simulink model "nov11"  (R2014a)
settings: Solver=ode45  StartTime=0.0  StopTime=30  FixedStep=0.00001  RelTol=1e-12
values from neighbouring files (symbols this model uses):
  m = [1 t0 (t0)^2 (t0)^3;0 1 (2*(t0)^2) (3*(t0)^2);1 tf (tf)^2 (tf)^3;0 1 (2*(tf)^2) (3*(tf)^2)]    [ControlCinematico.m]    (also in untitled3.m = [1 0 0 0 0 0;0 1 0 0 0 0;0 0 2 0 0 0;1 tf tf^2 tf^3 tf^4 tf^)
libraries: mblibv1 x15
settings Model: Creator=sebastian  LastModifiedBy=root
settings DataIOCC: SignalLoggingSaveFormat=ModelDataLogs
settings DebuggingCC: UnderspecifiedInitializationDetection=Classic  MultiTaskDSMMsg=warning  MultiTaskCondExecSysMsg=none  StateNameClashWarn=warning
settings RTWCC: IncludeERTFirstTime=on
settings SimMechanicsCC: VisOnUpdateDiagram=on  VisDuringSimulation=on

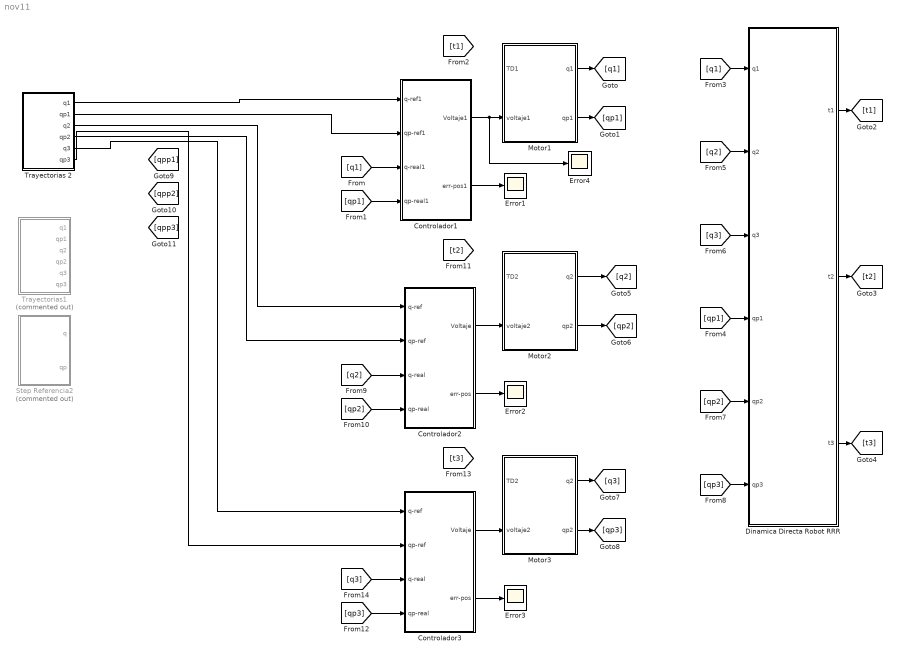
== system nov11 ==
  Controlador1 : Subsystem
  Controlador2 : Subsystem
  Controlador3 : Subsystem
  Dinamica Directa Robot RRR : Subsystem
  Error{1..4} (4 alike) : Scope
      Error1 settings: TimeRange=0.000199999999999978  YMin=-470000  YMax=-455000  SaveName=ScopeData4
      Error2 settings: YMin=0.3178  YMax=0.3188
      Error3 settings: YMin=0.675  YMax=1  SaveName=ScopeData5
      Error4 settings: YMin=-0.12  YMax=0  SaveName=ScopeData12
  Motor1 : Subsystem
  Motor2 : Subsystem
  Motor3 : Subsystem
  Step Referencia2 : Subsystem  Commented=on
  Trayectorias 2 : Subsystem
  Trayectorias1 : Subsystem  Commented=on
  wires:
  Controlador1/1(Voltaje1) -> Error4/1, Motor1/2(voltaje1)
  Controlador1/2(err-pos1) -> Error1/1
  Motor1/1(q1) -> [q1]
  Motor1/2(qp1) -> [qp1]
  Dinamica Directa Robot RRR/1(t1) -> [t1]
  [q1] -> Controlador1/3(q-real1)
  [qp1] -> Controlador1/4(qp-real1)
  [q1] -> Dinamica Directa Robot RRR/1(q1)
  [qp1] -> Dinamica Directa Robot RRR/4(qp1)
  [q2] -> Dinamica Directa Robot RRR/2(q2)
  [q3] -> Dinamica Directa Robot RRR/3(q3)
  [qp2] -> Dinamica Directa Robot RRR/5(qp2)
  [qp3] -> Dinamica Directa Robot RRR/6(qp3)
  Dinamica Directa Robot RRR/2(t2) -> [t2]
  Dinamica Directa Robot RRR/3(t3) -> [t3]
  Controlador2/1(Voltaje) -> Motor2/2(voltaje2)
  Controlador2/2(err-pos) -> Error2/1
  [q2] -> Controlador2/3(q-real)
  [qp2] -> Controlador2/4(qp-real)
  Controlador3/1(Voltaje) -> Motor3/2(voltaje2)
  Controlador3/2(err-pos) -> Error3/1
  Motor3/1(q2) -> [q3]
  Motor3/2(qp2) -> [qp3]
  [q3] -> Controlador3/3(q-real)
  [qp3] -> Controlador3/4(qp-real)
  Motor2/1(q2) -> [q2]
  Motor2/2(qp2) -> [qp2]
  Trayectorias 2/1(q1) -> Controlador1/1(q-ref1)
  Trayectorias 2/2(qp1) -> Controlador1/2(qp-ref1)
  Trayectorias 2/3(q2) -> Controlador2/1(q-ref)
  Trayectorias 2/4(qp2) -> Controlador2/2(qp-ref)
  Trayectorias 2/5(q3) -> Controlador3/1(q-ref)
  Trayectorias 2/6(qp3) -> Controlador3/2(qp-ref)

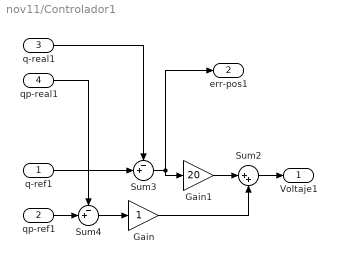
== system nov11/Controlador1 ==
  q-ref1 : Inport
  qp-ref1 : Inport  Port=2
  q-real1 : Inport  Port=3
  qp-real1 : Inport  Port=4
  Gain : Gain
  Gain1 : Gain  Gain=20
  Sum2 : Sum  Inputs=|++
  Sum3 : Sum  Inputs=-+|
  Sum4 : Sum  Inputs=-+|
  Voltaje1 : Outport
  err-pos1 : Outport  Port=2
  wires:
  Gain1/1 -> Sum2/1
  Gain/1 -> Sum2/2
  Sum4/1 -> Gain/1
  Sum2/1 -> Voltaje1/1
  q-ref1/1 -> Sum3/2
  qp-ref1/1 -> Sum4/2
  q-real1/1 -> Sum3/1
  qp-real1/1 -> Sum4/1
  Sum3/1 -> Gain1/1, err-pos1/1

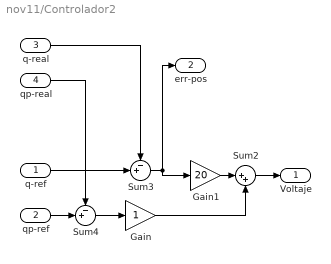
== system nov11/Controlador2 ==
  q-ref : Inport
  qp-ref : Inport  Port=2
  q-real : Inport  Port=3
  qp-real : Inport  Port=4
  Gain : Gain
  Gain1 : Gain  Gain=20
  Sum2 : Sum  Inputs=|++
  Sum3 : Sum  Inputs=-+|
  Sum4 : Sum  Inputs=-+|
  Voltaje : Outport
  err-pos : Outport  Port=2
  wires:
  Gain1/1 -> Sum2/1
  Gain/1 -> Sum2/2
  Sum4/1 -> Gain/1
  Sum2/1 -> Voltaje/1
  q-ref/1 -> Sum3/2
  qp-ref/1 -> Sum4/2
  q-real/1 -> Sum3/1
  qp-real/1 -> Sum4/1
  Sum3/1 -> Gain1/1, err-pos/1

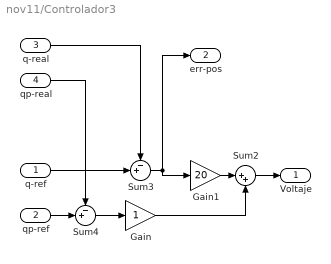
== system nov11/Controlador3 ==
  q-ref : Inport
  qp-ref : Inport  Port=2
  q-real : Inport  Port=3
  qp-real : Inport  Port=4
  Gain : Gain
  Gain1 : Gain  Gain=20
  Sum2 : Sum  Inputs=|++
  Sum3 : Sum  Inputs=-+|
  Sum4 : Sum  Inputs=-+|
  Voltaje : Outport
  err-pos : Outport  Port=2
  wires:
  Gain1/1 -> Sum2/1
  Gain/1 -> Sum2/2
  Sum4/1 -> Gain/1
  Sum2/1 -> Voltaje/1
  q-ref/1 -> Sum3/2
  qp-ref/1 -> Sum4/2
  q-real/1 -> Sum3/1
  qp-real/1 -> Sum4/1
  Sum3/1 -> Gain1/1, err-pos/1

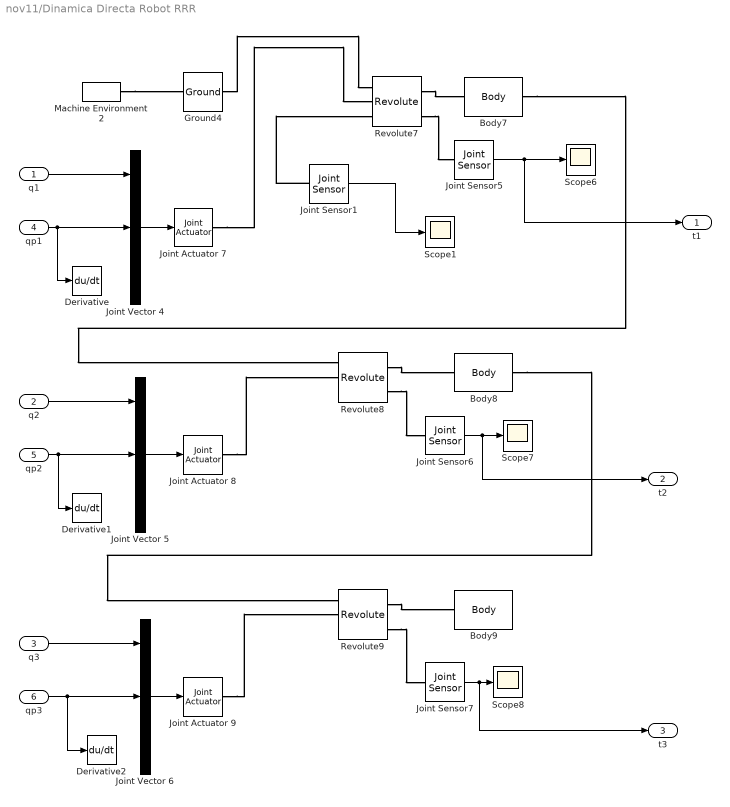
== system nov11/Dinamica Directa Robot RRR ==
  q1 : Inport
  q2 : Inport  Port=2
  q3 : Inport  Port=3
  qp1 : Inport  Port=4
  qp2 : Inport  Port=5
  qp3 : Inport  Port=6
  Body7 : mblibv1/Bodies/Body  LConnTagsString=CS1  RConnTagsString=CS2  UpdateFromCAD=off  DialogClass=MechanicalBodyBlock  Mass=1  MassUnits=kg  InertiaUnits=kg*m^2  Inertia=[0 0 0;0 0 0;0 0 33.3333]  Shape=Cylinder  ShapeDims=[1 1]  ShapeUnits=m  ShapeUse=false  Density=1  DensityUnits=kg/m^3  DensityUse=false  GraphicsMode=MACHINE_DEFAULT  BodyColorSelMode=COLORPALETTE  BodyColor=[0 1 0]  AttachedToCS=CG  CG=Left$CG$[0 10 0]$WORLD$WORLD$m$[0 0 0]$Euler X-Y-Z$deg$WORLD$false$none  WorkingFrames=Left$CS1$[0 0 0]$World$World$m$[0 0 0]$Euler X-Y-Z$deg$WORLD$true$none#Right$CS2$[0 20 0]$World$World$m$[0 0 0]$Euler X-Y-Z$deg$WORLD$true$none  CGPos=[0 10 0]  CGRot=[0 0 0]  CS0Pos=[]  CS0Rot=[]  CS1Pos=[0 0 0]  CS1Rot=[0 0 0]  CS2Pos=[0 20 0]  CS2Rot=[0 0 0]  CS3Pos=[]  CS3Rot=[]  CS4Pos=[]  CS4Rot=[]  CS5Pos=[]  CS5Rot=[]  CS6Pos=[]  CS6Rot=[]  CS7Pos=[]  CS7Rot=[]  CS8Pos=[]  CS8Rot=[]  CS9Pos=[]  CS9Rot=[]  CS10Pos=[]  CS10Rot=[]  CS11Pos=[]  CS11Rot=[]  CS12Pos=[]  CS12Rot=[]  CS13Pos=[]  CS13Rot=[]  CS14Pos=[]  CS14Rot=[]  CS15Pos=[]  CS15Rot=[]  CS16Pos=[]  CS16Rot=[]  CS17Pos=[]  CS17Rot=[]  CS18Pos=[]  CS18Rot=[]  CS19Pos=[]  CS19Rot=[]  CS20Pos=[]  CS20Rot=[]
  Body8 : mblibv1/Bodies/Body  LConnTagsString=CS1  RConnTagsString=CS2  UpdateFromCAD=off  DialogClass=MechanicalBodyBlock  Mass=1  MassUnits=kg  InertiaUnits=kg*m^2  Inertia=[0 0 0;0 0 0;0 0 33.3333]  Shape=Cylinder  ShapeDims=[1 1]  ShapeUnits=m  ShapeUse=false  Density=1  DensityUnits=kg/m^3  DensityUse=false  GraphicsMode=MACHINE_DEFAULT  BodyColorSelMode=COLORPALETTE  BodyColor=[0 1 0]  AttachedToCS=CG  CG=Left$CG$[10 20 0]$WORLD$WORLD$m$[0 0 0]$Euler X-Y-Z$deg$WORLD$false$none  WorkingFrames=Left$CS1$[0 20 0]$World$World$m$[0 0 0]$Euler X-Y-Z$deg$WORLD$true$none#Right$CS2$[20 20 0]$World$World$m$[0 0 0]$Euler X-Y-Z$deg$WORLD$true$none  CGPos=[10 20 0]  CGRot=[0 0 0]  CS0Pos=[]  CS0Rot=[]  CS1Pos=[0 20 0]  CS1Rot=[0 0 0]  CS2Pos=[20 20 0]  CS2Rot=[0 0 0]  CS3Pos=[]  CS3Rot=[]  CS4Pos=[]  CS4Rot=[]  CS5Pos=[]  CS5Rot=[]  CS6Pos=[]  CS6Rot=[]  CS7Pos=[]  CS7Rot=[]  CS8Pos=[]  CS8Rot=[]  CS9Pos=[]  CS9Rot=[]  CS10Pos=[]  CS10Rot=[]  CS11Pos=[]  CS11Rot=[]  CS12Pos=[]  CS12Rot=[]  CS13Pos=[]  CS13Rot=[]  CS14Pos=[]  CS14Rot=[]  CS15Pos=[]  CS15Rot=[]  CS16Pos=[]  CS16Rot=[]  CS17Pos=[]  CS17Rot=[]  CS18Pos=[]  CS18Rot=[]  CS19Pos=[]  CS19Rot=[]  CS20Pos=[]  CS20Rot=[]
  Body9 : mblibv1/Bodies/Body  LConnTagsString=CS1  RConnTagsString=CS2  UpdateFromCAD=off  DialogClass=MechanicalBodyBlock  Mass=1  MassUnits=kg  InertiaUnits=kg*m^2  Inertia=[0 0 0;0 0 0;0 0 8.3333]  Shape=Cylinder  ShapeDims=[1 1]  ShapeUnits=m  ShapeUse=false  Density=1  DensityUnits=kg/m^3  DensityUse=false  GraphicsMode=MACHINE_DEFAULT  BodyColorSelMode=COLORPALETTE  BodyColor=[0 1 0]  AttachedToCS=CG  CG=Left$CG$[20 15 0]$WORLD$WORLD$m$[0 0 0]$Euler X-Y-Z$deg$WORLD$false$none  WorkingFrames=Left$CS1$[20 20 0]$World$World$m$[0 0 0]$Euler X-Y-Z$deg$WORLD$true$none#Right$CS2$[20 10 0]$World$World$m$[0 0 0]$Euler X-Y-Z$deg$WORLD$true$none  CGPos=[20 15 0]  CGRot=[0 0 0]  CS0Pos=[]  CS0Rot=[]  CS1Pos=[20 20 0]  CS1Rot=[0 0 0]  CS2Pos=[20 10 0]  CS2Rot=[0 0 0]  CS3Pos=[]  CS3Rot=[]  CS4Pos=[]  CS4Rot=[]  CS5Pos=[]  CS5Rot=[]  CS6Pos=[]  CS6Rot=[]  CS7Pos=[]  CS7Rot=[]  CS8Pos=[]  CS8Rot=[]  CS9Pos=[]  CS9Rot=[]  CS10Pos=[]  CS10Rot=[]  CS11Pos=[]  CS11Rot=[]  CS12Pos=[]  CS12Rot=[]  CS13Pos=[]  CS13Rot=[]  CS14Pos=[]  CS14Rot=[]  CS15Pos=[]  CS15Rot=[]  CS16Pos=[]  CS16Rot=[]  CS17Pos=[]  CS17Rot=[]  CS18Pos=[]  CS18Rot=[]  CS19Pos=[]  CS19Rot=[]  CS20Pos=[]  CS20Rot=[]
  Derivative : Derivative
  Derivative1 : Derivative
  Derivative2 : Derivative
  Ground4 : mblibv1/Bodies/Ground  UpdateFromCAD=off  LeftPortType=env  RightPortType=workingframe  PhysicalDomain=Mechanical  DialogClass=GroundBlock  CoordPosition=[0 0 0]  CoordPositionUnits=m  StateVectorMgrId=1  MachineId=[2 0]  ShowEnvPort=on  ParameterChecksum=[821500782, 2772552656, 1304883052, 3709367703]  TopologyChecksum=[4015144124, 1642793208, 2502497068, 3913265325]
  Joint Actuator 7 : mblibv1/Sensors &  Actuators/Joint Actuator  UpdateFromCAD=off  PhysicalDomain=Mechanical  PortType=blob  ActuationStyle=Motion  AngleUnits=rad  ArcVelocityUnits=rad/s  ArcAccelerationUnits=rad/s^2  CoordPositionUnits=m  VelocityUnits=m/s  AccelerationUnits=m/s^2  ForceUnits=N  TorqueUnits=N*m  ActiveIO=on  Width=3  DialogClass=MechanicalActuatorBlock  Primitive=R1  ReferenceFrame=Absolute (World)
  Joint Actuator 8 : mblibv1/Sensors &  Actuators/Joint Actuator  UpdateFromCAD=off  PhysicalDomain=Mechanical  PortType=blob  ActuationStyle=Motion  AngleUnits=rad  ArcVelocityUnits=rad/s  ArcAccelerationUnits=rad/s^2  CoordPositionUnits=m  VelocityUnits=m/s  AccelerationUnits=m/s^2  ForceUnits=N  TorqueUnits=N*m  ActiveIO=on  Width=3  DialogClass=MechanicalActuatorBlock  Primitive=R1  ReferenceFrame=Absolute (World)
  Joint Actuator 9 : mblibv1/Sensors &  Actuators/Joint Actuator  UpdateFromCAD=off  PhysicalDomain=Mechanical  PortType=blob  ActuationStyle=Motion  AngleUnits=rad  ArcVelocityUnits=rad/s  ArcAccelerationUnits=rad/s^2  CoordPositionUnits=m  VelocityUnits=m/s  AccelerationUnits=m/s^2  ForceUnits=N  TorqueUnits=N*m  ActiveIO=on  Width=3  DialogClass=MechanicalActuatorBlock  Primitive=R1  ReferenceFrame=Absolute (World)
  Joint Sensor1 : mblibv1/Sensors &  Actuators/Joint Sensor  UpdateFromCAD=off  PhysicalDomain=Mechanical  PortType=blob  Muxed=on  Pose=off  Angle=on  AngleUnits=rad  ArcVelocity=off  ArcVelocityUnits=deg/s  ArcAcceleration=off  ArcAccelerationUnits=deg/s^2  CoordPosition=on  CoordPositionUnits=m  Velocity=off  VelocityUnits=m/s  Acceleration=off  AccelerationUnits=m/s^2  Quaternion=on  QuaternionDT=off  QuaternionDDT=off  QuaternionUnits=off  OutputVector=[1]  ActiveIO=on  Width=1  DialogClass=MechanicalSensorBlock  Primitive=R1  Force=off  ForceUnits=N  Torque=off  TorqueUnits=N*m  ReferenceFrame=Absolute (World)  ReactionSensedSide=Follower  ReactionReferenceFrame=Absolute (World)  ReactionForce=off  ReactionForceUnits=N  ReactionMoment=off  ReactionMomentUnits=N*m
  Joint Sensor5 : mblibv1/Sensors &  Actuators/Joint Sensor  UpdateFromCAD=off  PhysicalDomain=Mechanical  PortType=blob  Muxed=on  Pose=off  Angle=off  AngleUnits=deg  ArcVelocity=off  ArcVelocityUnits=deg/s  ArcAcceleration=off  ArcAccelerationUnits=deg/s^2  CoordPosition=on  CoordPositionUnits=m  Velocity=off  VelocityUnits=m/s  Acceleration=off  AccelerationUnits=m/s^2  Quaternion=on  QuaternionDT=off  QuaternionDDT=off  QuaternionUnits=off  OutputVector=[1]  ActiveIO=on  Width=1  DialogClass=MechanicalSensorBlock  Primitive=R1  Force=off  ForceUnits=N  Torque=on  TorqueUnits=N*m  ReferenceFrame=Absolute (World)  ReactionSensedSide=Follower  ReactionReferenceFrame=Absolute (World)  ReactionForce=off  ReactionForceUnits=N  ReactionMoment=off  ReactionMomentUnits=N*m
  Joint Sensor6 : mblibv1/Sensors &  Actuators/Joint Sensor  UpdateFromCAD=off  PhysicalDomain=Mechanical  PortType=blob  Muxed=on  Pose=off  Angle=off  AngleUnits=deg  ArcVelocity=off  ArcVelocityUnits=deg/s  ArcAcceleration=off  ArcAccelerationUnits=deg/s^2  CoordPosition=on  CoordPositionUnits=m  Velocity=off  VelocityUnits=m/s  Acceleration=off  AccelerationUnits=m/s^2  Quaternion=on  QuaternionDT=off  QuaternionDDT=off  QuaternionUnits=off  OutputVector=[1]  ActiveIO=on  Width=1  DialogClass=MechanicalSensorBlock  Primitive=R1  Force=off  ForceUnits=N  Torque=on  TorqueUnits=N*m  ReferenceFrame=Absolute (World)  ReactionSensedSide=Follower  ReactionReferenceFrame=Absolute (World)  ReactionForce=off  ReactionForceUnits=N  ReactionMoment=off  ReactionMomentUnits=N*m
  Joint Sensor7 : mblibv1/Sensors &  Actuators/Joint Sensor  UpdateFromCAD=off  PhysicalDomain=Mechanical  PortType=blob  Muxed=on  Pose=off  Angle=off  AngleUnits=deg  ArcVelocity=off  ArcVelocityUnits=deg/s  ArcAcceleration=off  ArcAccelerationUnits=deg/s^2  CoordPosition=on  CoordPositionUnits=m  Velocity=off  VelocityUnits=m/s  Acceleration=off  AccelerationUnits=m/s^2  Quaternion=on  QuaternionDT=off  QuaternionDDT=off  QuaternionUnits=off  OutputVector=[1]  ActiveIO=on  Width=1  DialogClass=MechanicalSensorBlock  Primitive=R1  Force=off  ForceUnits=N  Torque=on  TorqueUnits=N*m  ReferenceFrame=Absolute (World)  ReactionSensedSide=Follower  ReactionReferenceFrame=Absolute (World)  ReactionForce=off  ReactionForceUnits=N  ReactionMoment=off  ReactionMomentUnits=N*m
  Joint Vector 4 : Concatenate  NumInputs=3
  Joint Vector 5 : Concatenate  NumInputs=3
  Joint Vector 6 : Concatenate  NumInputs=3
  Machine Environment2 : mblibv1/Bodies/Machine Environment  PortType=env  PhysicalDomain=Mechanical  DialogTemplateClass=MECH.MachineEnvironment  SyncWhenCopied=off  Gravity=[0 0 0]  GravityUnits=m/s^2  GravityAsSignal=off  Dimensionality=Auto-detect  AnalysisType=Inverse dynamics  LinearAssemblyTolerance=1e-3  LinearAssemblyToleranceUnits=m  AngularAssemblyTolerance=1e-3  AngularAssemblyToleranceUnits=rad  ConstraintSolverType=Stabilizing  ConstraintRelTolerance=1e-4  ConstraintAbsTolerance=1e-4  UseRobustSingularityHandling=off  RedundancyAnalysisToleranceType=Automatically select tolerance  RedundancyAnalysisTolerance=1e-14  StatePerturbationType=Fixed  PerturbationSize=1e-5  VisualizeMachine=on  BodyVisualizationType=Use model default body geometries  BodyColorSelMode=Use model default  DefaultBodyColor=[1 0 0]
  Revolute7 : mblibv1/Joints/Revolute  LConnTagsString=__newl0|SA1|SA2  RConnTagsString=__newr0|SA1  UpdateFromCAD=off  NumSAPorts=3  CutJoint=off  MarkAsCut=off  Primitives=prismatic  PrimitiveProps=R1$World$[0 0 1]$revolute  DialogClass=JointBlock  R1Axis=[0 0 1]
  Revolute8 : mblibv1/Joints/Revolute  LConnTagsString=__newl0|SA1|SA2  RConnTagsString=__newr0|SA1  UpdateFromCAD=off  NumSAPorts=3  CutJoint=off  MarkAsCut=off  Primitives=prismatic  PrimitiveProps=R1$World$[0 0 1]$revolute  DialogClass=JointBlock  R1Axis=[0 0 1]
  Revolute9 : mblibv1/Joints/Revolute  LConnTagsString=__newl0|SA1|SA2  RConnTagsString=__newr0|SA1  UpdateFromCAD=off  NumSAPorts=3  CutJoint=off  MarkAsCut=off  Primitives=prismatic  PrimitiveProps=R1$World$[0 0 1]$revolute  DialogClass=JointBlock  R1Axis=[0 0 1]
  Scope{1,6..8} (4 alike) : Scope
      Scope1 settings: TimeRange=30  YMin=-2.525e+08  YMax=-2.35e+08  SaveName=ScopeData13
      Scope6 settings: TimeRange=30  YMin=-2.525e+08  YMax=-2.35e+08  SaveName=ScopeData9
      Scope7 settings: TimeRange=30  SaveName=ScopeData10
      Scope8 settings: TimeRange=30  SaveName=ScopeData11
  t1 : Outport
  t2 : Outport  Port=2
  t3 : Outport  Port=3
  wires:
  Joint Vector 5/1 -> Joint Actuator 8/1
  Joint Vector 4/1 -> Joint Actuator 7/1
  Joint Vector 6/1 -> Joint Actuator 9/1
  Joint Sensor5/1 -> t1/1, Scope6/1
  Joint Sensor7/1 -> t3/1, Scope8/1
  Joint Sensor6/1 -> t2/1, Scope7/1
  q1/1 -> Joint Vector 4/1
  q2/1 -> Joint Vector 5/1
  q3/1 -> Joint Vector 6/1
  qp1/1 -> Derivative/1, Joint Vector 4/2
  qp2/1 -> Derivative1/1, Joint Vector 5/2
  qp3/1 -> Derivative2/1, Joint Vector 6/2
  Joint Sensor1/1 -> Scope1/1
  connections:
  Revolute9/RConn1 -- Body9/LConn1
  Body7/RConn1 -- Revolute8/LConn1
  Body8/RConn1 -- Revolute9/LConn1
  Revolute8/RConn2 -- Joint Sensor6/LConn1
  Joint Actuator 8/RConn1 -- Revolute8/LConn2
  Revolute8/RConn1 -- Body8/LConn1
  Ground4/RConn1 -- Revolute7/LConn1
  Revolute7/RConn1 -- Body7/LConn1
  Revolute7/RConn2 -- Joint Sensor5/LConn1
  Revolute9/RConn2 -- Joint Sensor7/LConn1
  Joint Actuator 9/RConn1 -- Revolute9/LConn2
  Machine Environment2/RConn1 -- Ground4/LConn1
  Joint Actuator 7/RConn1 -- Revolute7/LConn2
  Joint Sensor1/LConn1 -- Revolute7/LConn3

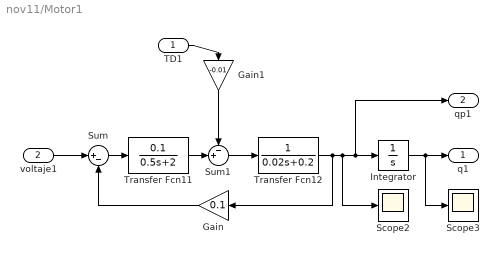
== system nov11/Motor1 ==
  TD1 : Inport
  voltaje1 : Inport  Port=2
  Gain : Gain  Gain=0.1
  Gain1 : Gain  Gain=-0.01
  Integrator : Integrator
  Scope2 : Scope
  Scope3 : Scope
      settings: SaveName=ScopeData3
  Sum : Sum  Inputs=|+-
  Sum1 : Sum  Inputs=-+|
  Transfer Fcn11 : TransferFcn  Numerator=[0.1]  Denominator=[0.5 2]
  Transfer Fcn12 : TransferFcn  Denominator=[0.02 0.2]
  q1 : Outport
  qp1 : Outport  Port=2
  wires:
  Sum/1 -> Transfer Fcn11/1
  Sum1/1 -> Transfer Fcn12/1
  Transfer Fcn11/1 -> Sum1/2
  Gain/1 -> Sum/2
  Transfer Fcn12/1 -> qp1/1, Integrator/1, Scope2/1, Gain/1
  Integrator/1 -> q1/1, Scope3/1
  voltaje1/1 -> Sum/1
  TD1/1 -> Gain1/1
  Gain1/1 -> Sum1/1

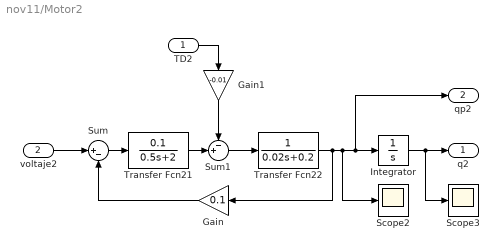
== system nov11/Motor2 ==
  TD2 : Inport
  voltaje2 : Inport  Port=2
  Gain : Gain  Gain=0.1
  Gain1 : Gain  Gain=-0.01
  Integrator : Integrator
  Scope2 : Scope
  Scope3 : Scope
      settings: SaveName=ScopeData3
  Sum : Sum  Inputs=|+-
  Sum1 : Sum  Inputs=-+|
  Transfer Fcn21 : TransferFcn  Numerator=[0.1]  Denominator=[0.5 2]
  Transfer Fcn22 : TransferFcn  Denominator=[0.02 0.2]
  q2 : Outport
  qp2 : Outport  Port=2
  wires:
  Sum/1 -> Transfer Fcn21/1
  Sum1/1 -> Transfer Fcn22/1
  Transfer Fcn21/1 -> Sum1/2
  Gain/1 -> Sum/2
  Transfer Fcn22/1 -> qp2/1, Integrator/1, Scope2/1, Gain/1
  Integrator/1 -> q2/1, Scope3/1
  voltaje2/1 -> Sum/1
  TD2/1 -> Gain1/1
  Gain1/1 -> Sum1/1

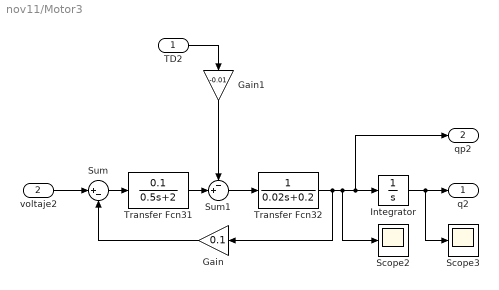
== system nov11/Motor3 ==
  TD2 : Inport
  voltaje2 : Inport  Port=2
  Gain : Gain  Gain=0.1
  Gain1 : Gain  Gain=-0.01
  Integrator : Integrator
  Scope2 : Scope
  Scope3 : Scope
      settings: SaveName=ScopeData3
  Sum : Sum  Inputs=|+-
  Sum1 : Sum  Inputs=-+|
  Transfer Fcn31 : TransferFcn  Numerator=[0.1]  Denominator=[0.5 2]
  Transfer Fcn32 : TransferFcn  Denominator=[0.02 0.2]
  q2 : Outport
  qp2 : Outport  Port=2
  wires:
  Sum/1 -> Transfer Fcn31/1
  Sum1/1 -> Transfer Fcn32/1
  Transfer Fcn31/1 -> Sum1/2
  Gain/1 -> Sum/2
  Transfer Fcn32/1 -> qp2/1, Integrator/1, Scope2/1, Gain/1
  Integrator/1 -> q2/1, Scope3/1
  voltaje2/1 -> Sum/1
  TD2/1 -> Gain1/1
  Gain1/1 -> Sum1/1

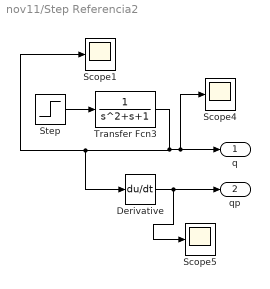
== system nov11/Step Referencia2 ==
  Derivative : Derivative
  Scope1 : Scope
      settings: SaveName=ScopeData6
  Scope4 : Scope
      settings: SaveName=ScopeData7
  Scope5 : Scope
      settings: SaveName=ScopeData8
  Step : Step  After=0.1  SampleTime=0
  Transfer Fcn3 : TransferFcn  Denominator=[1 1 1]
  q : Outport
  qp : Outport  Port=2
  wires:
  Step/1 -> Transfer Fcn3/1
  Transfer Fcn3/1 -> q/1, Scope4/1, Derivative/1, Scope1/1
  Derivative/1 -> Scope5/1, qp/1

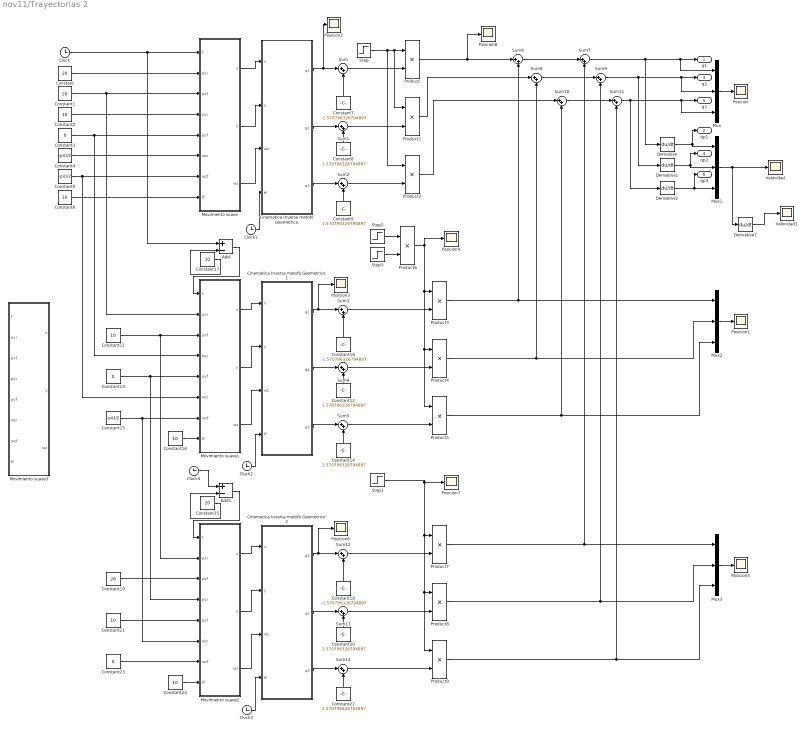
== system nov11/Trayectorias 2 ==
  Add : Sum  Inputs=+-
  Add1 : Sum  Inputs=+-
  "Cinematica Inversa metofo Geometrico " : MATLAB Function  TreatAsAtomicUnit=on
  Cinematica Inversa metofo Geometrico 1 : MATLAB Function  TreatAsAtomicUnit=on
  Cinematica Inversa metofo Geometrico 2 : MATLAB Function  TreatAsAtomicUnit=on
  Clock{,1..4} (5 alike) : Clock
  Constant{,1,19,25} (4 alike) : Constant  Value=20
  Constant10 : Constant  Value=-1.570796326794897
  Constant{2,6,11,16..17,21,24} (7 alike) : Constant  Value=10
  Constant{8..9,12,14,20,22} (6 alike) : Constant  Value=1.570796326794897
  Constant13 : Constant  Value=0
  Constant15 : Constant  Value=-pi()/2
  Constant18 : Constant  Value=-1.570796326794897
  Constant23 : Constant  Value=0
  Constant3 : Constant  Value=0
  Constant4 : Constant  Value=-pi()/2
  Constant5 : Constant  Value=-pi()/2
  Constant7 : Constant  Value=-1.570796326794897
  Derivative{,1..3} (4 alike) : Derivative
  Movimiento suave : MATLAB Function  TreatAsAtomicUnit=on
  Movimiento suave1 : MATLAB Function  TreatAsAtomicUnit=on
  Movimiento suave2 : MATLAB Function  TreatAsAtomicUnit=on
  Movimiento suave3 : MATLAB Function  TreatAsAtomicUnit=on
  Mux{,1..3} (4 alike) : Mux  Inputs=3
  Posicion{,1..8} (9 alike) : Scope
      Posicion settings: TimeRange=1.736204576043068  YMin=-0.9624756335282649  YMax=0.6817738791423005  SaveName=ScopeData14
      Posicion1 settings: SaveName=ScopeData16
      Posicion2 settings: SaveName=ScopeData17
      Posicion3 settings: YMin=1.25221  YMax=1.38403  SaveName=ScopeData18
      Posicion4 settings: SaveName=ScopeData19
      Posicion5 settings: SaveName=ScopeData20
      Posicion6 settings: SaveName=ScopeData21
      Posicion7 settings: SaveName=ScopeData22
      Posicion8 settings: SaveName=ScopeData23
  Product{,1..9} (10 alike) : Product
  Step : Step  Time=10  Before=1  After=0  SampleTime=0
  Step1 : Step  Time=20  SampleTime=0
  Step2 : Step  Time=10  SampleTime=0
  Step3 : Step  Time=20  Before=1  After=0  SampleTime=0
  Sum{,1..14} (15 alike) : Sum  Inputs=|++
  Velocidad : Scope
      settings: SaveName=ScopeData15
  Velocidad1 : Scope
      settings: SaveName=ScopeData24
  q1 : Outport
  qp1 : Outport  Port=2
  q2 : Outport  Port=3
  qp2 : Outport  Port=4
  q3 : Outport  Port=5
  qp3 : Outport  Port=6
  wires:
  Mux/1 -> Posicion/1
  Derivative/1 -> Mux1/1, qp1/1
  Derivative2/1 -> qp3/1, Mux1/3
  Derivative1/1 -> Mux1/2, qp2/1
  Constant/1 -> Movimiento suave/2(pxi)
  Constant2/1 -> Movimiento suave/4(pyi)
  Constant6/1 -> Movimiento suave/8(tf)
  Movimiento suave/3(wz) -> "Cinematica Inversa metofo Geometrico "/3(wz)
  Movimiento suave/1(x) -> "Cinematica Inversa metofo Geometrico "/1(x)
  Movimiento suave/2(y) -> "Cinematica Inversa metofo Geometrico "/2(y)
  Constant4/1 -> Movimiento suave/6(wzi)
  "Cinematica Inversa metofo Geometrico "/2(q2) -> Sum1/1
  "Cinematica Inversa metofo Geometrico "/3(q3) -> Sum2/1
  Constant8/1 -> Sum1/2
  Constant7/1 -> Sum/2
  "Cinematica Inversa metofo Geometrico "/1(q1) -> Posicion2/1, Sum/1
  Constant9/1 -> Sum2/2
  Clock/1 -> Movimiento suave/1(t), Add/1
  Constant1/1 -> Movimiento suave1/2(pxi), Movimiento suave/3(pxf)
  Constant3/1 -> Movimiento suave1/4(pyi), Movimiento suave/5(pyf)
  Constant13/1 -> Movimiento suave2/4(pyi), Movimiento suave1/5(pyf)
  Constant15/1 -> Movimiento suave2/6(wzi), Movimiento suave1/7(wzf)
  Constant16/1 -> Movimiento suave1/8(tf)
  Constant5/1 -> Movimiento suave1/6(wzi), Movimiento suave/7(wzf)
  Step/1 -> Product2/1, Product1/1, Product/1
  Cinematica Inversa metofo Geometrico 1/2(q2) -> Sum4/1
  Cinematica Inversa metofo Geometrico 1/3(q3) -> Sum5/1
  Constant12/1 -> Sum4/2
  Constant10/1 -> Sum3/2
  Cinematica Inversa metofo Geometrico 1/1(q1) -> Posicion3/1, Sum3/1
  Constant14/1 -> Sum5/2
  Sum2/1 -> Product2/2
  Sum1/1 -> Product1/2
  Sum/1 -> Product/2
  Sum6/1 -> Sum7/1
  Sum7/1 -> Mux/1, q1/1, Derivative/1
  Sum8/1 -> Sum9/1
  Sum9/1 -> Mux/2, q2/1, Derivative1/1
  Sum10/1 -> Sum11/1
  Sum11/1 -> Mux/3, q3/1, Derivative2/1
  Product/1 -> Posicion8/1, Sum6/1
  Product1/1 -> Sum8/1
  Product2/1 -> Sum10/1
  Sum3/1 -> Product3/2
  Sum4/1 -> Product4/2
  Sum5/1 -> Product5/2
  Mux2/1 -> Posicion1/1
  Product4/1 -> Sum8/2, Mux2/2
  Product5/1 -> Sum10/2, Mux2/3
  Add/1 -> Movimiento suave1/1(t)
  Constant17/1 -> Add/2
  Clock1/1 -> "Cinematica Inversa metofo Geometrico "/4(tf)
  Clock2/1 -> Cinematica Inversa metofo Geometrico 1/4(tf)
  Product3/1 -> Sum6/2, Mux2/1
  Step2/1 -> Product6/1
  Step3/1 -> Product6/2
  Product6/1 -> Product5/1, Product4/1, Product3/1, Posicion4/1
  Constant19/1 -> Movimiento suave2/3(pxf)
  Constant21/1 -> Movimiento suave2/5(pyf)
  Constant23/1 -> Movimiento suave2/7(wzf)
  Constant24/1 -> Movimiento suave2/8(tf)
  Movimiento suave2/3(wz) -> Cinematica Inversa metofo Geometrico 2/3(wz)
  Movimiento suave2/1(x) -> Cinematica Inversa metofo Geometrico 2/1(x)
  Movimiento suave2/2(y) -> Cinematica Inversa metofo Geometrico 2/2(y)
  Cinematica Inversa metofo Geometrico 2/2(q2) -> Sum13/1
  Cinematica Inversa metofo Geometrico 2/3(q3) -> Sum14/1
  Constant20/1 -> Sum13/2
  Constant18/1 -> Sum12/2
  Cinematica Inversa metofo Geometrico 2/1(q1) -> Posicion6/1, Sum12/1
  Constant22/1 -> Sum14/2
  Sum12/1 -> Product7/2
  Sum13/1 -> Product8/2
  Sum14/1 -> Product9/2
  Mux3/1 -> Posicion5/1
  Product8/1 -> Sum9/2, Mux3/2
  Product9/1 -> Mux3/3, Sum11/2
  Add1/1 -> Movimiento suave2/1(t)
  Constant25/1 -> Add1/2
  Clock3/1 -> Cinematica Inversa metofo Geometrico 2/4(tf)
  Product7/1 -> Sum7/2, Mux3/1
  Step1/1 -> Product9/1, Product8/1, Product7/1, Posicion7/1
  Constant11/1 -> Movimiento suave2/2(pxi), Movimiento suave1/3(pxf)
  Clock4/1 -> Add1/1
  Movimiento suave1/1(x) -> Cinematica Inversa metofo Geometrico 1/1(x)
  Movimiento suave1/2(y) -> Cinematica Inversa metofo Geometrico 1/2(y)
  Movimiento suave1/3(wz) -> Cinematica Inversa metofo Geometrico 1/3(wz)
  Mux1/1 -> Derivative3/1, Velocidad/1
  Derivative3/1 -> Velocidad1/1

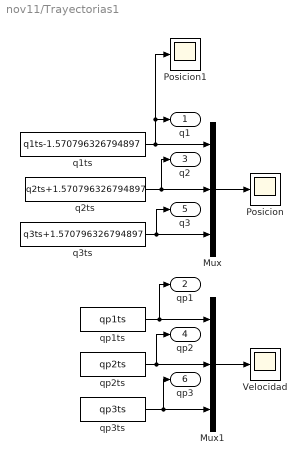
== system nov11/Trayectorias1 ==
  Mux : Mux  Inputs=3
  Mux1 : Mux  Inputs=3
  Posicion : Scope
      settings: SaveName=ScopeData14
  Posicion1 : Scope
      settings: SaveName=ScopeData2
  Velocidad : Scope
      settings: SaveName=ScopeData15
  q1ts : FromWorkspace  VariableName=q1ts-1.570796326794897  SampleTime=0  OutputAfterFinalValue=Holding final value
  q2ts : FromWorkspace  VariableName=q2ts+1.570796326794897  SampleTime=0  OutputAfterFinalValue=Holding final value
  q3ts : FromWorkspace  VariableName=q3ts+1.570796326794897  SampleTime=0  OutputAfterFinalValue=Holding final value
  qp1ts : FromWorkspace  VariableName=qp1ts  SampleTime=0  OutputAfterFinalValue=Setting to zero
  qp2ts : FromWorkspace  VariableName=qp2ts  SampleTime=0  OutputAfterFinalValue=Setting to zero
  qp3ts : FromWorkspace  VariableName=qp3ts  SampleTime=0  OutputAfterFinalValue=Setting to zero
  q1 : Outport
  qp1 : Outport  Port=2
  q2 : Outport  Port=3
  qp2 : Outport  Port=4
  q3 : Outport  Port=5
  qp3 : Outport  Port=6
  wires:
  Mux/1 -> Posicion/1
  q1ts/1 -> Mux/1, Posicion1/1, q1/1
  q3ts/1 -> q3/1, Mux/3
  q2ts/1 -> q2/1, Mux/2
  Mux1/1 -> Velocidad/1
  qp1ts/1 -> qp1/1, Mux1/1
  qp3ts/1 -> qp3/1, Mux1/3
  qp2ts/1 -> qp2/1, Mux1/2

== matlab function nov11/Trayectorias 2/Cinematica Inversa metofo Geometrico  ==
  data: x input; y input; wz input; q1 output; q2 output; q3 output; tf input
function [q1,q2,q3]= fcn(x,y,wz,tf)
l3=10;
l1=20;
l2=20;

    if tf > 10
    q1=0;
    q2=0;
    q3=0;
    else
xw = x-l3*cos(wz);
yw = y-l3*sin(wz);

q2 = -acos((xw^2 + yw^2 - l1^2 - l2^2)/(2*l1*l2));
q1 = asin((l2*sin(-q2))/(sqrt(xw^2 + yw^2))) + atan(yw/xw);

q3= wz-q1-q2;

    end

== matlab function nov11/Trayectorias 2/Movimiento suave ==
  data: t input; x output; pxi input; pxf input; pyi input; pyf input; wzi input; wzf input; y output; wz output; tf input
function [x,y,wz]= fcn(t,pxi,pxf,pyi,pyf,wzi,wzf,tf)

a0x = pxi;
a1x = 0; %velocidad inicial
a2x = 0; %aceleracion inicial
a3x = (10*(pxf-pxi))/tf^3;
a4x = -(15*(pxf-pxi))/tf^4;
a5x = (6*(pxf-pxi))/tf^5;
x = a0x + a1x*t + a2x*t^2 + a3x*t^3 + a4x*t^4 + a5x*t^5;
a0y = pyi;
a1y = 0; %velocidad inicial
a2y = 0; %aceleracion inicial
a3y = (10*(pyf-pyi))/tf^3;
a4y = -(15*(pyf-pyi))/tf^4;
a5y = (6*(pyf-pyi))/tf^5;
y = a0y + a1y*t + a2y*t^2 + a3y*t^3 + a4y*t^4 + a5y*t^5;
a0wz = wzi;
a1wz = 0; %velocidad inicial
a2wz = 0; %aceleracion inicial
a3wz = (10*(wzf-wzi))/tf^3;
a4wz = -(15*(wzf-wzi))/tf^4;
a5wz = (6*(wzf-wzi))/tf^5;
wz = a0wz + a1wz*t + a2wz*t^2 + a3wz*t^3 + a4wz*t^4 + a5wz*t^5;

== matlab function nov11/Trayectorias 2/Cinematica Inversa metofo Geometrico 1 ==
  data: x input; y input; wz input; q1 output; q2 output; q3 output; tf input
function [q1,q2,q3]= fcn(x,y,wz,tf)
l3=10;
l1=20;
l2=20;

    if tf < 10
    q1=0;
    q2=0;
    q3=0;
    
    elseif tf > 20
     q1=0;
    q2=0;
    q3=0;
        
    else
        
    xw = x-l3*cos(wz);
    yw = y-l3*sin(wz);

    q2 = -acos((xw^2 + yw^2 - l1^2 - l2^2)/(2*l1*l2));
    q1 = asin((l2*sin(-q2))/(sqrt(xw^2 + yw^2))) + atan(yw/xw);

    q3= wz-q1-q2;

    end

== matlab function nov11/Trayectorias 2/Movimiento suave1 ==
  data: t input; x output; pxi input; pxf input; pyi input; pyf input; wzi input; wzf input; y output; wz output; tf input
function [x,y,wz]= fcn(t,pxi,pxf,pyi,pyf,wzi,wzf,tf)

a0x = pxi;
a1x = 0; %velocidad inicial
a2x = 0; %aceleracion inicial
a3x = (10*(pxf-pxi))/tf^3;
a4x = -(15*(pxf-pxi))/tf^4;
a5x = (6*(pxf-pxi))/tf^5;
x = a0x + a1x*t + a2x*t^2 + a3x*t^3 + a4x*t^4 + a5x*t^5;
a0y = pyi;
a1y = 0; %velocidad inicial
a2y = 0; %aceleracion inicial
a3y = (10*(pyf-pyi))/tf^3;
a4y = -(15*(pyf-pyi))/tf^4;
a5y = (6*(pyf-pyi))/tf^5;
y = a0y + a1y*t + a2y*t^2 + a3y*t^3 + a4y*t^4 + a5y*t^5;
a0wz = wzi;
a1wz = 0; %velocidad inicial
a2wz = 0; %aceleracion inicial
a3wz = (10*(wzf-wzi))/tf^3;
a4wz = -(15*(wzf-wzi))/tf^4;
a5wz = (6*(wzf-wzi))/tf^5;
wz = a0wz + a1wz*t + a2wz*t^2 + a3wz*t^3 + a4wz*t^4 + a5wz*t^5;

== matlab function nov11/Trayectorias 2/Cinematica Inversa metofo Geometrico 2 ==
  data: x input; y input; wz input; q1 output; q2 output; q3 output; tf input
function [q1,q2,q3]= fcn(x,y,wz,tf)
l3=10;
l1=20;
l2=20;

    if tf < 20
    q1=0;
    q2=0;
    q3=0;
    
    elseif tf > 30
     q1=0;
    q2=0;
    q3=0;
        
    else
        
    xw = x-l3*cos(wz);
    yw = y-l3*sin(wz);

    q2 = -acos((xw^2 + yw^2 - l1^2 - l2^2)/(2*l1*l2));
    q1 = asin((l2*sin(-q2))/(sqrt(xw^2 + yw^2))) + atan(yw/xw);

    q3= wz-q1-q2;

    end

== matlab function nov11/Trayectorias 2/Movimiento suave2 ==
  data: t input; x output; pxi input; pxf input; pyi input; pyf input; wzi input; wzf input; y output; wz output; tf input
function [x,y,wz]= fcn(t,pxi,pxf,pyi,pyf,wzi,wzf,tf)

a0x = pxi;
a1x = 0; %velocidad inicial
a2x = 0; %aceleracion inicial
a3x = (10*(pxf-pxi))/tf^3;
a4x = -(15*(pxf-pxi))/tf^4;
a5x = (6*(pxf-pxi))/tf^5;
x = a0x + a1x*t + a2x*t^2 + a3x*t^3 + a4x*t^4 + a5x*t^5;
a0y = pyi;
a1y = 0; %velocidad inicial
a2y = 0; %aceleracion inicial
a3y = (10*(pyf-pyi))/tf^3;
a4y = -(15*(pyf-pyi))/tf^4;
a5y = (6*(pyf-pyi))/tf^5;
y = a0y + a1y*t + a2y*t^2 + a3y*t^3 + a4y*t^4 + a5y*t^5;
a0wz = wzi;
a1wz = 0; %velocidad inicial
a2wz = 0; %aceleracion inicial
a3wz = (10*(wzf-wzi))/tf^3;
a4wz = -(15*(wzf-wzi))/tf^4;
a5wz = (6*(wzf-wzi))/tf^5;
wz = a0wz + a1wz*t + a2wz*t^2 + a3wz*t^3 + a4wz*t^4 + a5wz*t^5;

== matlab function nov11/Trayectorias 2/Movimiento suave3 ==
  data: t input; x output; pxi input; pxf input; pyi input; pyf input; wzi input; wzf input; y output; wz output; tf input
function [x,y,wz]= fcn(t,pxi,pxf,pyi,pyf,wzi,wzf,tf)

x = pxi + ((3*(pxf-pxi))/(tf^2))*t^2 - ((2*(pxf-pxi))/(tf^3))*t^3;
y = pyi + ((3*(pyf-pyi))/(tf^2))*t^2 - ((2*(pyf-pyi))/(tf^3))*t^3;
wz = wzi + ((3*(wzf-wzi))/(tf^2))*t^2 - ((2*(wzf-wzi))/(tf^3))*t^3;
